simulink model "transmisor"  (R2025b)
settings: Solver=FixedStepDiscrete  StartTime=0.0  StopTime=6000  FixedStep=1/3312  RelTol=1e-3
libraries: commcnvcod2 x2, commdigbbndpm3 x2, commfilt2 x2, commchan3 x1
settings Model: VariantFading=off  Creator=karolpalechor  LastModifiedBy=briyi

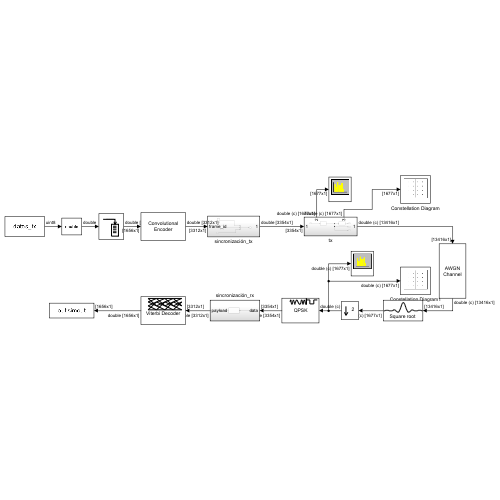
[thumbnail: Simulink's stored preview of the top-level diagram]
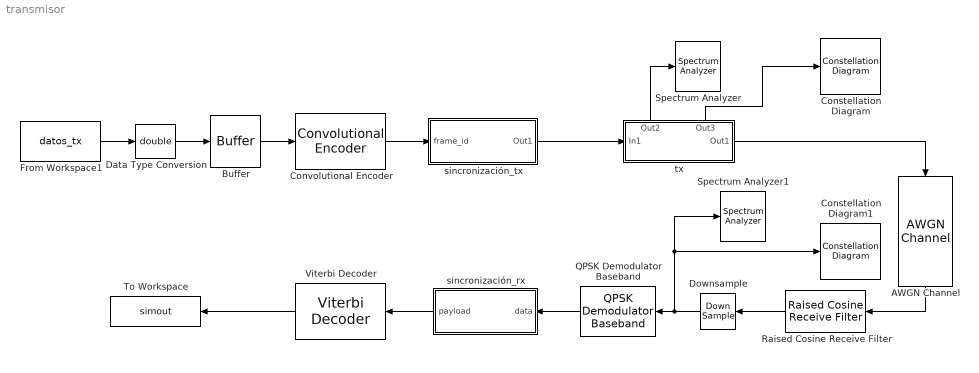
== system transmisor ==
  AWGN Channel : commchan3/AWGN Channel  LegacyMode=off  NoiseMethod="Signal to noise ratio  (Eb/No)"  noiseMode="Signal to noise ratio  (SNR)"  EbNo=20  EsNo=10  SNR=10  BitsPerSymbol=2  SignalPower=1  SpecifySymbolPeriod=on  SamplesPerSymbol=1  SymbolPeriod=1  VarianceSource=Parameter  Variance=1  RandomStream=Global stream  Seed=67  SimulateUsing=Code generation
  Buffer : Buffer  N=1656  OutputFrames=off
  Constellation Diagram : ConstellationDiagram  WindowPosition=[2.000000,50.000000,766.000000,785.000000,]  Visible=on  ScopeFrameLocation=window
  Constellation Diagram1 : ConstellationDiagram  WindowPosition=[770.000000,50.000000,766.000000,785.000000,]  Visible=on  ScopeFrameLocation=window
  Convolutional Encoder : commcnvcod2/Convolutional Encoder  trellis=poly2trellis(7, [171 133])  opMode=Continuous  DelayedResetAction=off  hasIniStPort=off  hasFinStPort=off  usePuncVector=off  punctureVector=[1; 1; 0; 1; 0; 1]  reset=Unused parameter value
  Data Type Conversion : DataTypeConversion  OutDataTypeStr=double  SaturateOnIntegerOverflow=off  RndMeth=Floor
  Downsample : DownSample  AllowArbitraryFixedInput=on
  From Workspace1 : FromWorkspace  VariableName=datos_tx  OutDataTypeStr=uint8  SampleTime=1/1656  Interpolate=off  ZeroCross=off  OutputAfterFinalValue=Holding final value
  QPSK Demodulator Baseband : commdigbbndpm3/QPSK Demodulator Baseband  OutType=Bit  DecType=Hard decision  VarSource=Dialog  Variance=1  Dec=Gray  Ph=pi/4  outDtype1=Inherit via internal rule  outDtype2=Inherit via internal rule  derotateFactorWordLen=16  derotateFactorDataTypeStr=Inherit: Same word length as input  derotateFactorLastDataTypeStr=Inherit: Same word length as input
  Raised Cosine Receive Filter : commfilt2/Raised Cosine Receive Filter  filtType=Square root  R=0.25  filtSpan=10  N=8  downFactor=8  downOffset=0  filterGain=1  InputProcessing=Columns as channels (frame based)  RateOptions=Enforce single-rate processing  framing=Mute  checkCoeff=off  variableName=rcRxFilt  currentFiltSpan=10  D=5  inputOffset=0  sampMode=Mute  saveAsFlag=0  rateMode=Downsampling  checkGain=Normalized  launchFVT=on  roundingMode=Floor  overflowMode=off  coeffDataTypeStr=Inherit: Same word length as input  coeffMin=[]  coeffMax=[]  coeffLastDataTypeStr=Inherit: Same word length as input  accumDataTypeStr=Inherit: Same as product output  accumLastDataTypeStr=Inherit: Same as product output  outputDataTypeStr=Inherit: Same as accumulator  outputMin=[]  outputMax=[]  outputLastDataTypeStr=Inherit: Same as accumulator
  Spectrum Analyzer : SpectrumAnalyzer  WindowPosition=[729.000000,11.000000,800.000000,500.000000,]  Visible=on  ScopeFrameLocation=window  WindowInvariantSamplesPerUpdate=on  YLimits=[-45.8018 38.2721]
  Spectrum Analyzer1 : SpectrumAnalyzer  WindowPosition=[532.000000,259.000000,800.000000,500.000000,]  Visible=on  ScopeFrameLocation=window  WindowInvariantSamplesPerUpdate=on  YLimits=[1.1944 32.8743]
  To Workspace : ToWorkspace  VariableName=simout  SampleTime=-1
      settings: Save2DSignal=2-D array (concatenate along first dimension)
  Viterbi Decoder : commcnvcod2/Viterbi Decoder  trellis=poly2trellis(7,[171 133])  isPunctured=off  punctureVector=[1; 1; 0; 1; 0; 1]  erasures=off  dectype=Hard decision  nsdecb=3  runSigValErrCheck=off  tbdepth=34  opmode=Continuous  reset=off  delayedResetAction=off  smWordLength=16  outDataType=Inherit via internal rule
  sincronización_rx : Subsystem
  sincronización_tx : Subsystem
  tx : Subsystem
      settings: PortSchema="{\"entries\":[{\"content\":{\"sides\":[{\"content\":{\"connectorIds\":[\"In1\"]},\"type\":\"ConnectorPlacement.EquallySpacedRectSide\",\"uuid\":\"b164cc83-15cb-4dc1-a3f1-a1e4e105ed67\"},{\"content\":{\"connectorIds\":[\"Out1\"],\"side\":\"RIGHT\"},\"type\":\"ConnectorPlacement.EquallySpacedRectSide\",\"uuid\":\"e1a365a7-8c38-48c2-9d5a-857c3ea336b3\"},{\"content\":{\"connectorIds\":[\"Out2\",\"Out3\"],\"side\":\"TOP\"},\"type\":\"ConnectorPlacement.EquallySpacedRectSide\",\"uuid\":\"54bb274e-9742-4539-9706-175e2d4a2cfd\"}]},\"type\":\"ConnectorPlacement.EquallySpacedConnector\",\"uuid\":\"ceaa24bc-0563-41ba-9ac2-0c1f5fceca54\"}],\"packageUris\":[\"http://schema.mathworks.com/mf0/Connector/R2020b\"],\"version\":\"1.0\"}"
  wires:
  QPSK Demodulator Baseband/1 -> sincronización_rx/1(data)
  sincronización_tx/1(Out1) -> tx/1(In1)
  tx/1(Out1) -> AWGN Channel/1
  Buffer/1 -> Convolutional Encoder/1
  From Workspace1/1 -> Data Type Conversion/1
  Data Type Conversion/1 -> Buffer/1
  Viterbi Decoder/1 -> To Workspace/1
  Convolutional Encoder/1 -> sincronización_tx/1(frame_id)
  sincronización_rx/1(payload) -> Viterbi Decoder/1
  tx/2(Out2) -> Spectrum Analyzer/1
  tx/3(Out3) -> Constellation Diagram/1
  Raised Cosine Receive Filter/1 -> Downsample/1
  AWGN Channel/1 -> Raised Cosine Receive Filter/1
  Downsample/1 -> Constellation Diagram1/1, Spectrum Analyzer1/1, QPSK Demodulator Baseband/1

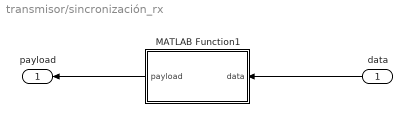
== system transmisor/sincronización_rx ==
  data : Inport
  MATLAB Function1 : MATLAB Function  TreatAsAtomicUnit=on
  payload : Outport  OutDataTypeStr=double
  wires:
  MATLAB Function1/1(payload) -> payload/1
  data/1 -> MATLAB Function1/1(data)

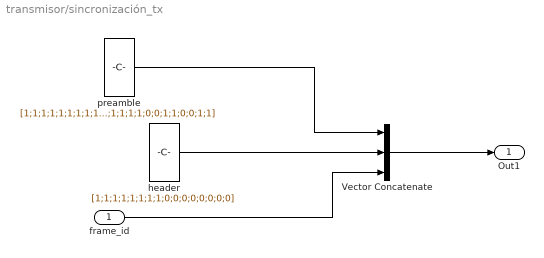
== system transmisor/sincronización_tx ==
  frame_id : Inport
  Vector Concatenate : Concatenate  NumInputs=3
  header : Constant  Value=[1;1;1;1;1;1;1;1;0;0;0;0;0;0;0;0]  VectorParams1D=off  OutDataTypeStr=double  SampleTime=-1
  preamble : Constant  Value=[1;1;1;1;1;1;1;1;1;1;0;0;0;0;1;1;1;1;0;0;1;1;0;0;1;1]  VectorParams1D=off  OutDataTypeStr=double  SampleTime=-1
  Out1 : Outport
  wires:
  Vector Concatenate/1 -> Out1/1
  preamble/1 -> Vector Concatenate/1
  frame_id/1 -> Vector Concatenate/3
  header/1 -> Vector Concatenate/2

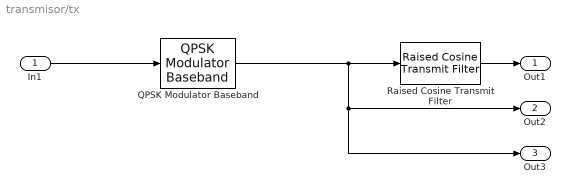
== system transmisor/tx ==
  In1 : Inport
  QPSK Modulator Baseband : commdigbbndpm3/QPSK Modulator Baseband  InType=Bit  Enc=Gray  Ph=pi/4  outDtype=Inherit via back propagation  outWordLen=16  outUDDataType=sfix(16)  outFracLenMode=Best precision  outFracLen=15  outDataTypeStr=Inherit: Inherit via back propagation  outLastDataTypeStr=Inherit: Inherit via back propagation
  Raised Cosine Transmit Filter : commfilt2/Raised Cosine Transmit Filter  filtType=Square root  R=0.25  filtSpan=10  N=8  filterGain=1  InputProcessing=Columns as channels (frame based)  RateOptions=Enforce single-rate processing  framing=Mute  checkCoeff=off  variableName=rcTxFilt  checkGain=Normalized  sampMode=Mute  saveAsFlag=0  currentFiltSpan=10  D=(10)/2  launchFVT=on  roundingMode=Floor  overflowMode=off  coeffDataTypeStr=Inherit: Same word length as input  coeffMin=[]  coeffMax=[]  coeffLastDataTypeStr=Inherit: Same word length as input  outputDataTypeStr=Inherit: Same as accumulator  outputMin=[]  outputMax=[]  outputLastDataTypeStr=Inherit: Same as accumulator
  Out1 : Outport
  Out2 : Outport  Port=2
  Out3 : Outport  Port=3
  wires:
  QPSK Modulator Baseband/1 -> Out3/1, Out2/1, Raised Cosine Transmit Filter/1
  Raised Cosine Transmit Filter/1 -> Out1/1
  In1/1 -> QPSK Modulator Baseband/1

== matlab function transmisor/sincronización_rx/MATLAB Function1 ==
  data: data input; payload output
function payload = extract(data)
%#codegen
payload_len = int32(3312);
payload     = zeros(payload_len, 1, 'double');
sync_len    = int32(42);
data_len    = int32(length(data));

for j = int32(1):payload_len
    pos = sync_len + j;
    if pos <= data_len
        payload(j) = data(pos);
    end
end

end
